simulink model "test05"  (R2021a)
settings: Solver=VariableStepAuto  StartTime=0.0  StopTime=5  RelTol=1e-3
libraries: HORTISIM x6
settings Model: Creator=djoroya  LastModifiedBy=djoroya
settings DebuggingCC: UnconnectedInputMsg=none  UnconnectedOutputMsg=none  UnconnectedLineMsg=none

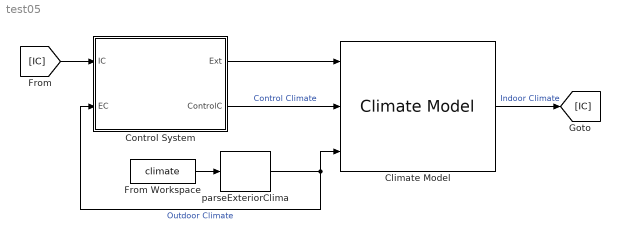
== system test05 ==
  Climate Model : HORTISIM/Climate/Models/Climate Model  hour0=0  G0=[0.05 0.0007]  T0=[273 273 273 273]+15  H=7  A_f=3200  A_c=3200  minWindows=0.01  lam_s=[2.5000 0.8500]  c_s=[1081 1081]  l_s=[0.1000 0.1000]  rhod_s=[2600 2500]  int_air_speed=0.5  alpha_i=0.1  alpha_c=0.05  tau_c=0.9  alpha_f=0.1  d_c=1.5  cd_c=8736  T_ss=285.15
      settings: SourceProductName=Horti Simulator
  Control System : Subsystem
  From Workspace : FromWorkspace  VariableName=climate
  parseExteriorClima : HORTISIM/Other  Functions/parseExteriorClima  SystemSampleTime=-1  VariantActivationTime=update diagram  Latency=0  AutoFrameSizeCalculation=off
      settings: SourceProductName=Horti Simulator
  wires:
  From Workspace/1 -> parseExteriorClima/1
  parseExteriorClima/1 -> Climate Model/3, Control System/2(EC)  "Outdoor Climate"
  Climate Model/1 -> [IC]  "Indoor Climate"
  Control System/2(ControlC) -> Climate Model/2  "Control Climate"
  [IC] -> Control System/1(IC)
  Control System/1(Ext) -> Climate Model/1

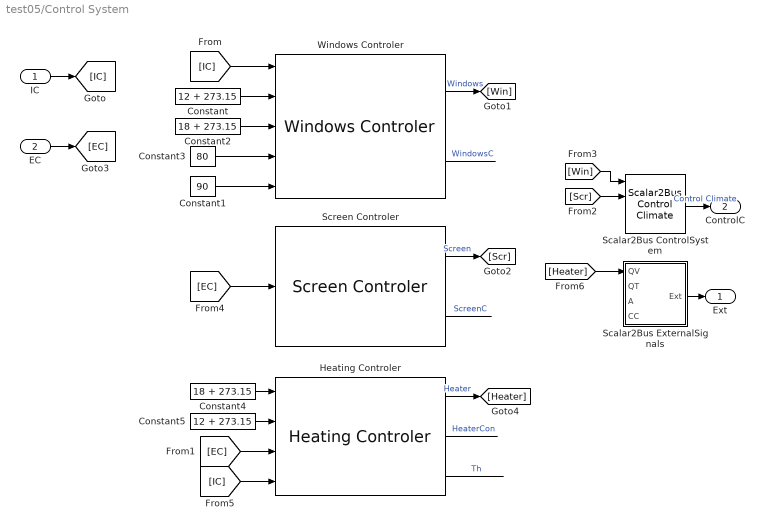
== system test05/Control System ==
  IC : Inport
  EC : Inport  Port=2
  Constant : Constant  Value=12 + 273.15
  Constant1 : Constant  Value=90
  Constant2 : Constant  Value=18 + 273.15
  Constant3 : Constant  Value=80
  Constant4 : Constant  Value=18 + 273.15
  Constant5 : Constant  Value=12 + 273.15
  Heating Controler : HORTISIM/Climate/Controls/Heating Controler  T=288  power=1000e3  A_e=6e-4  A_i=6e-4  c=1e-8
      settings: SourceProductName=Horti Simulator
  Scalar2Bus ControlSystem : HORTISIM/Other  Functions/Scalar2Bus  Control Climate  SystemSampleTime=-1  VariantActivationTime=update diagram  Latency=0  AutoFrameSizeCalculation=off
      settings: SourceProductName=Horti Simulator
  Scalar2Bus ExternalSignals : Subsystem
  Screen Controler : HORTISIM/Climate/Controls/Screen Controler  Radthreshold=200  velocity=0.33333  Power=0  gamma_max=0.3  beta=0.1
      settings: SourceProductName=Horti Simulator
  Windows Controler : HORTISIM/Climate/Controls/Windows Controler  Power=100  max_night=10  tau=600  RadThreshold=10  AR=10
      settings: SourceProductName=Horti Simulator
  Ext : Outport
  ControlC : Outport  Port=2
  wires:
  Constant2/1 -> Windows Controler/3
  Constant3/1 -> Windows Controler/4
  Windows Controler/2 -> ?  "WindowsC"
  Constant1/1 -> Windows Controler/5
  Constant/1 -> Windows Controler/2
  IC/1 -> [IC]
  [IC] -> Windows Controler/1
  Windows Controler/1 -> [Win]  "Windows"
  Screen Controler/1 -> [Scr]  "Screen"
  [Scr] -> Scalar2Bus ControlSystem/2
  [Win] -> Scalar2Bus ControlSystem/1
  Scalar2Bus ControlSystem/1 -> ControlC/1  "Control Climate"
  EC/1 -> [EC]
  [EC] -> Screen Controler/1
  Screen Controler/2 -> ?  "ScreenC"
  [EC] -> Heating Controler/3
  [IC] -> Heating Controler/4
  Constant4/1 -> Heating Controler/1
  Constant5/1 -> Heating Controler/2
  Heating Controler/1 -> [Heater]  "Heater"
  [Heater] -> Scalar2Bus ExternalSignals/1(QV)
  Scalar2Bus ExternalSignals/1(Ext) -> Ext/1
  Heating Controler/3 -> ?  "Th"
  Heating Controler/2 -> ?  "HeaterCon"

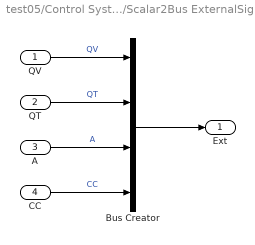
== system test05/Control System/Scalar2Bus ExternalSignals ==
  QV : Inport
  QT : Inport  Port=2
  A : Inport  Port=3
  CC : Inport  Port=4
  Bus Creator : BusCreator  Inputs=4
  Ext : Outport
  wires:
  QT/1 -> Bus Creator/2  "QT"
  QV/1 -> Bus Creator/1  "QV"
  A/1 -> Bus Creator/3  "A"
  CC/1 -> Bus Creator/4  "CC"
  Bus Creator/1 -> Ext/1
